simulink model "DC_CONTROL"  (R2019b)
settings: Solver=VariableStepAuto  StartTime=0.0  StopTime=20.0  RelTol=1e-3
undefined symbols (not defined in the file): Gv, ki, Tv
settings Model: Creator=simone  LastModifiedBy=simone
settings SolverCC: ZeroCrossAlgorithm=Adaptive
settings DebuggingCC: IgnoredZcDiagnostic=none

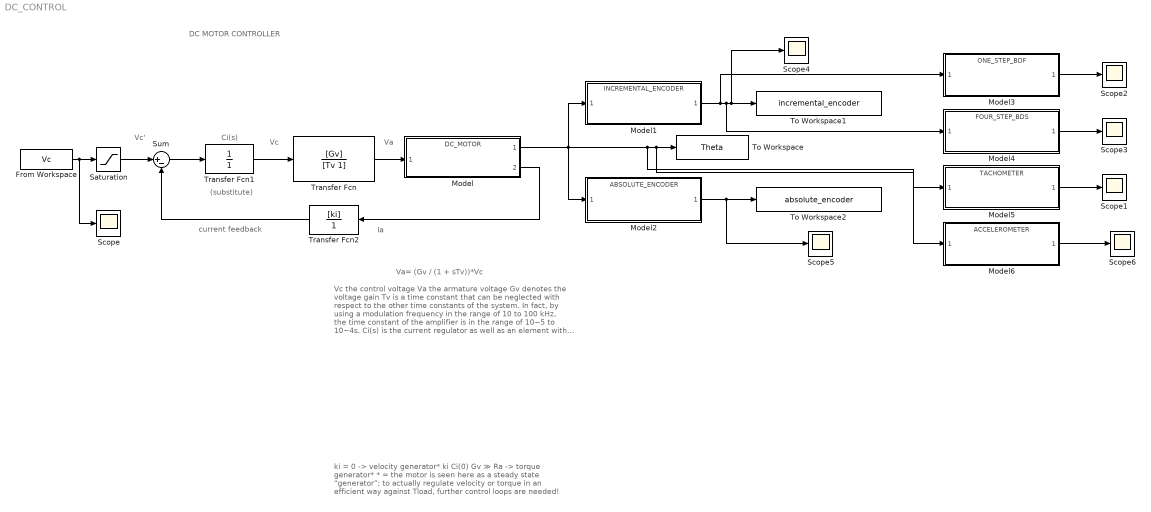
== system DC_CONTROL ==
  note: ki = 0 -> velocity generator*
      | ki Ci(0) Gv ≫ Ra -> torque generator*
      |
      | * = the motor is seen here as a steady state “generator”;
      | to actually regulate velocity or torque in an efficient way
      | against Tload, further control loops are needed!
  note: (substitute)
  note: current feedback
  note: Vc the control voltage
      |
      | Va the armature voltage
      |
      | Gv denotes the voltage gain
      |
      | Tv is a time constant that can be neglected with respect
      | to the other time constants of the system. In fact, by using
      | a modulation frequency in the range of 10 to 100 kHz,
      | the time constant of the amplifier is in the range of 10−5 to
      | 10−4s.
      |
      | Ci(s) is the current regulator as well as an element with a
      | nonlinear saturation characteristic. By means of a
      | suitable choice of the regulator Ci(s), the lag between
      | the current Ia and the voltage Vc′ can be reduced with
      | respect to the lag between Ia and Vc
      |
      | Vc′ the voltage plays the role of a current reference
      |
      | ki trasducer constant
  note: Va= (Gv / (1 + sTv))*Vc
  note: DC MOTOR CONTROLLER
  note: Ci(s)
  note: Vc'
  note: Va
  note: Vc
  note: Ia
  From Workspace : FromWorkspace  VariableName=Vc  SampleTime=0.01
  Model : ModelReference  ModelNameDialog=DC_MOTOR.slx  SimulationMode=Normal  ModelReferenceVersion=1.19
  Model1 : ModelReference  ModelNameDialog=INCREMENTAL_ENCODER.slx  SimulationMode=Normal  ModelReferenceVersion=1.21
  Model2 : ModelReference  ModelNameDialog=ABSOLUTE_ENCODER.slx  SimulationMode=Normal  ModelReferenceVersion=1.75
  Model3 : ModelReference  ModelNameDialog=ONE_STEP_BDF.slx  SimulationMode=Normal  ModelReferenceVersion=1.8
  Model4 : ModelReference  ModelNameDialog=FOUR_STEP_BDS.slx  SimulationMode=Normal  ModelReferenceVersion=1.3
  Model5 : ModelReference  ModelNameDialog=TACHOMETER.slx  SimulationMode=Normal  ModelReferenceVersion=1.9
  Model6 : ModelReference  ModelNameDialog=ACCELEROMETER.slx  SimulationMode=Normal  ModelReferenceVersion=1.4
  Saturation : Saturate  UpperLimit=1000  LowerLimit=-1000
  Scope{,1..6} (7 alike) : Scope
  Sum : Sum  Inputs=|+-
  To Workspace : ToWorkspace  VariableName=Theta  SaveFormat=Timeseries  SampleTime=-1
  To Workspace1 : ToWorkspace  VariableName=incremental_encoder  SaveFormat=Timeseries  SampleTime=-1
  To Workspace2 : ToWorkspace  VariableName=absolute_encoder  SaveFormat=Timeseries  SampleTime=-1
  Transfer Fcn : TransferFcn  Numerator=[Gv]  Denominator=[Tv 1]  ContinuousStateAttributes="\"\""
  Transfer Fcn1 : TransferFcn  Denominator=1  ContinuousStateAttributes="\""
  Transfer Fcn2 : TransferFcn  Numerator=[ki]  Denominator=[1]  ContinuousStateAttributes="\""
  wires:
  From Workspace/1 -> Scope/1, Saturation/1
  Saturation/1 -> Sum/1
  Transfer Fcn/1 -> Model/1
  Sum/1 -> Transfer Fcn1/1
  Transfer Fcn1/1 -> Transfer Fcn/1
  Model/2 -> Transfer Fcn2/1
  Transfer Fcn2/1 -> Sum/2
  Model2/1 -> Scope5/1, To Workspace2/1
  Model/1 -> Model1/1, Model6/1, Model5/1, To Workspace/1, Model2/1
  Model3/1 -> Scope2/1
  Model4/1 -> Scope3/1
  Model5/1 -> Scope1/1
  Model1/1 -> Model3/1, Model4/1, Scope4/1, To Workspace1/1
  Model6/1 -> Scope6/1
